simulink model "Actuador"  (R2022a)
settings: Solver=VariableStepAuto  StartTime=0.0  StopTime=10.0  RelTol=1e-3
undefined symbols (not defined in the file): kw
settings Model: Creator=juani  LastModifiedBy=juani
settings DebuggingCC: ModelReferenceExtraNoncontSigs=none

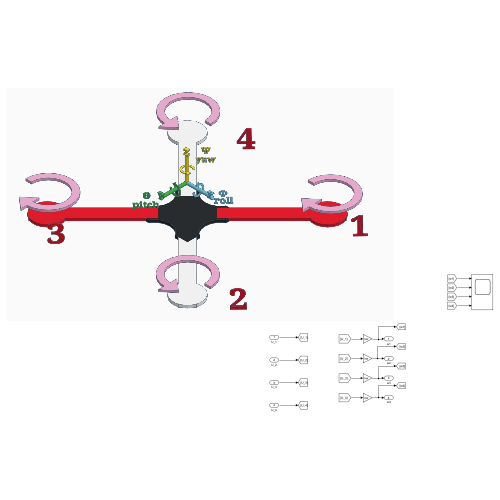
[thumbnail: Simulink's stored preview of the top-level diagram]
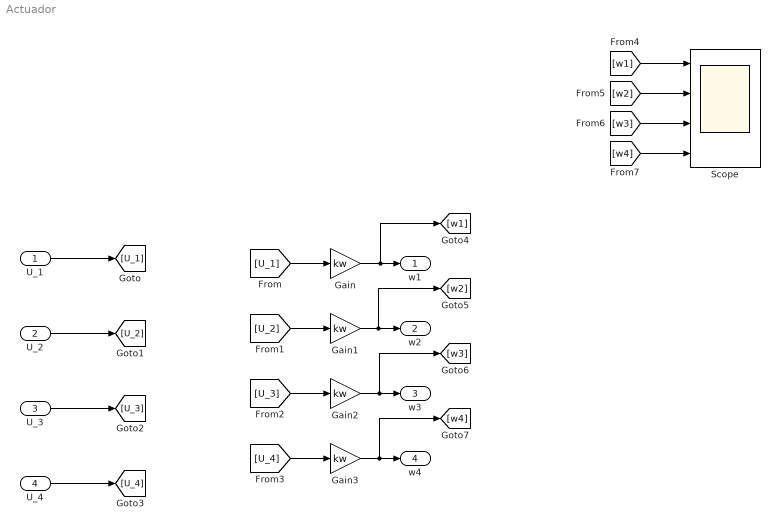
== system Actuador ==
  U_1 : Inport  SampleTime=0.001
  U_2 : Inport  Port=2
  U_3 : Inport  Port=3
  U_4 : Inport  Port=4
  Gain{,1..3} (4 alike) : Gain  Gain=kw
  Scope : Scope  NumInputPorts=4
  w1 : Outport
  w2 : Outport  Port=2
  w3 : Outport  Port=3
  w4 : Outport  Port=4
  wires:
  [U_2] -> Gain1/1
  [U_4] -> Gain3/1
  Gain1/1 -> [w2], w2/1
  U_1/1 -> [U_1]
  Gain/1 -> [w1], w1/1
  U_4/1 -> [U_4]
  [U_1] -> Gain/1
  U_3/1 -> [U_3]
  U_2/1 -> [U_2]
  Gain2/1 -> [w3], w3/1
  [w3] -> Scope/3
  [w2] -> Scope/2
  [w1] -> Scope/1
  [U_3] -> Gain2/1
  Gain3/1 -> [w4], w4/1
  [w4] -> Scope/4
